simulink model "chap9_1sim"  (Simulink 3.00)
settings: Solver=ode4  SolverMode=SingleTasking  StartTime=0.0  StopTime=3  FixedStep=0.001  RelTol=1e-3
settings Model: LastModifiedBy=liu

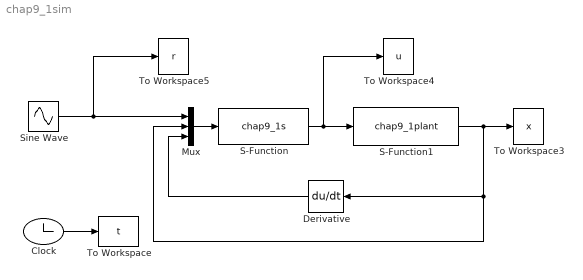
== system chap9_1sim ==
  Clock : Clock
  Derivative : Derivative  Orientation=left
  Mux : Mux  Inputs=3
  S-Function : S-Function  FunctionName=chap9_1s  PortCounts=[]  SFunctionModules=''
  S-Function1 : S-Function  FunctionName=chap9_1plant  PortCounts=[]  SFunctionModules=''
  Sine Wave : Sin  Amplitude=0.5  Frequency=2*pi  Phase=0  SampleTime=0
  To Workspace : ToWorkspace  VariableName=t  SampleTime=-1  SaveFormat=Matrix
  To Workspace3 : ToWorkspace  VariableName=x  SampleTime=-1  SaveFormat=Matrix
  To Workspace4 : ToWorkspace  VariableName=u  SampleTime=-1  SaveFormat=Matrix
  To Workspace5 : ToWorkspace  VariableName=r  SampleTime=-1  SaveFormat=Matrix
  wires:
  Mux/1 -> S-Function/1
  S-Function1/1 -> To Workspace3/1, Mux/2, Derivative/1
  Clock/1 -> To Workspace/1
  S-Function/1 -> S-Function1/1, To Workspace4/1
  Derivative/1 -> Mux/3
  Sine Wave/1 -> Mux/1, To Workspace5/1
